simulink model "shipp"  (R2016b)
settings: Solver=ode45  StartTime=0.0  StopTime=1000  RelTol=1e-3  EnableMultiTasking=on
values from neighbouring files (symbols this model uses):
  K = P_*data.Cd'*inv(data.Cd*P_*data.Cd'+data.R)    [Sfunctionshell.m]    (also in boatstuff.m = 0.1707)
  K_pd = 0.7647    [boatstuff.m]
  phi = 30    [boatstuff.m]
  T_d = T    (= 74.435)    [boatstuff.m]
  T_f = 8.391    [boatstuff.m]
libraries: simulink x4
settings Model: Creator=markh  LastModifiedBy=Kjetil
settings DataIOCC: LimitDataPoints=on  SaveFormat=Array  SignalLoggingSaveFormat=ModelDataLogs  SignalLoggingName=sigsOut
settings OptimizationCC: InitFltsAndDblsToZero=on  LifeSpan=inf
settings DebuggingCC: SaveWithParameterizedLinksMsg=none  UnderspecifiedInitializationDetection=Classic  MergeDetectMultiDrivingBlocksExec=none  SignalResolutionControl=TryResolveAllWithWarning  MultiTaskDSMMsg=warning  MultiTaskCondExecSysMsg=none  FcnCallInpInsideContextMsg=warning  StateNameClashWarn=warning  SFUnexpectedBacktrackingDiag=warning  SFNoUnconditionalDefaultTransitionDiag=warning  SFExecutionAtInitializationDiag=none
settings HardwareCC: ProdBitPerPointer=32  ProdBitPerSizeT=32  ProdBitPerPtrDiffT=32  ProdLargestAtomicFloat=None  ProdIntDivRoundTo=Undefined  ProdEndianess=Unspecified  ProdWordSize=32  ProdHWDeviceType=32-bit Generic  TargetUnknown=on
settings ModelReferenceCC: PropagateSignalLabelsOutOfModel=off
settings GRTTargetCC: TargetFcnLib=ansi_tfl_tmw.mat  TargetLangStandard=C89/C90 (ANSI)  GeneratePreprocessorConditionals=Disable all  CombineOutputUpdateFcns=off  GRTInterface=on
settings ConfigComp: CovMetricSettings=dw  CovHtmlReporting=on  CovSaveCumulativeToWorkspaceVar=on  CovSaveSingleToWorkspaceVar=on  CovExternalEMLEnable=off

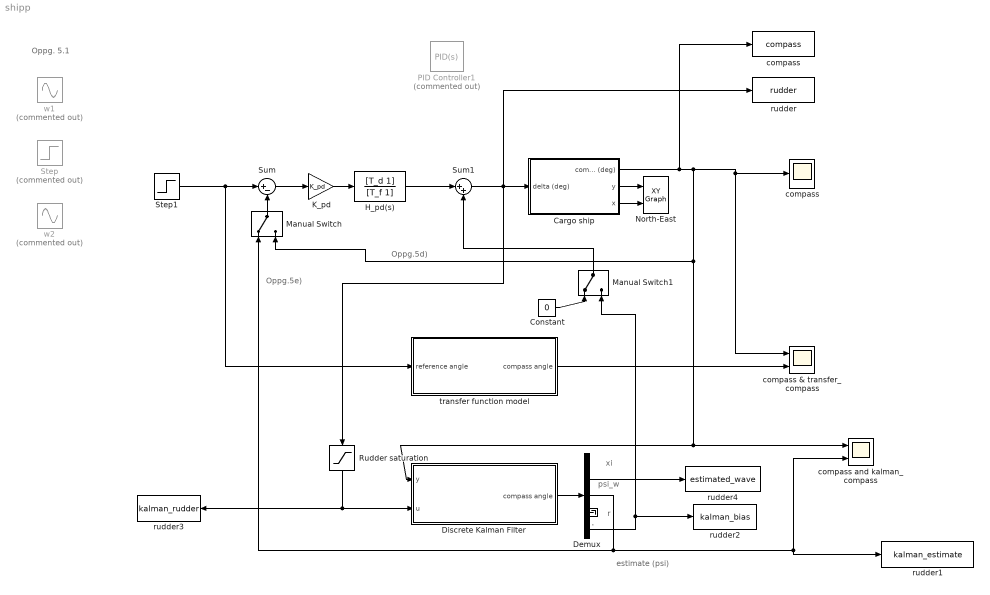
== system shipp ==
  note: Oppg.5d)
  note: Oppg.5e)
  note: r
  note: psi_w
  note: xi
  note: estimate (psi)
  note: Oppg. 5.1
  " H_pd(s)" : TransferFcn  Numerator=[T_d 1]  Denominator=[T_f 1]
  . : Terminator
  Cargo ship : Subsystem  mask(Simple shipmodel for a cargo ship){noise=on, current=on, logic=on}
      mask prompts: noise "measurement noise"; logic "waves"
      mask help:
      | Measurement noise:
      | 	checked = noise on
      | 	unchecked = noise off
      |
      | Current:
      | 	checked = current on
      | 	unchecked = current off
      |
      | Waves:
      | 	checked = waves on
      | 	unchecked = waves off
      |
      | Author: Jørgen Spjøtvold, 9/10-2003
      | TTK 4115 Linear system theory.
      | Modified by Jostein Bakkeheim 26/10-2006
  Constant : Constant  Value=0
  Demux : Demux  Outputs=5
  Discrete Kalman Filter : Subsystem
  K_pd : Gain  Gain=K_pd
  Manual Switch : ManualSwitch
  Manual Switch1 : ManualSwitch
  North-East : simulink/Sinks/XY Graph  xmin=-5000  xmax=5000  ymin=-5000  ymax=5000  st=-1
  PID Controller1 : simulink/Continuous/PID Controller  Commented=on  Controller=PID  TimeDomain=Continuous-time  SampleTime=-1  IntegratorMethod=Forward Euler  FilterMethod=Forward Euler  Form=Parallel  UseFilter=on  ControllerParametersSource=internal  P=0.0879832562005669  I=0.000147500393517768  D=7.30622580756413  N=0.0302786606051885  InitialConditionSource=internal  InitialConditionForIntegrator=0  InitialConditionForFilter=0  ExternalReset=none  LimitOutput=off  UpperSaturationLimit=inf  LowerSaturationLimit=-inf  LinearizeAsGain=on  AntiWindupMode=none  Kb=1  TrackingMode=off  Kt=1  PParamMin=[]  PParamMax=[]  IParamMin=[]  IParamMax=[]  DParamMin=[]  DParamMax=[]  NParamMin=[]  NParamMax=[]  KbParamMin=[]  KbParamMax=[]  KtParamMin=[]  KtParamMax=[]  POutMin=[]  POutMax=[]  IOutMin=[]  IOutMax=[]  DOutMin=[]  DOutMax=[]  NOutMin=[]  NOutMax=[]  KbOutMin=[]  KbOutMax=[]  KtOutMin=[]  KtOutMax=[]  IntegratorOutMin=[]  IntegratorOutMax=[]  FilterOutMin=[]  FilterOutMax=[]  SumOutMin=[]  SumOutMax=[]  SumI1OutMin=[]  SumI1OutMax=[]  SumI2OutMin=[]  SumI2OutMax=[]  SumI3OutMin=[]  SumI3OutMax=[]  SumDOutMin=[]  SumDOutMax=[]  SaturationOutMin=[]  SaturationOutMax=[]  IntegratorContinuousStateAttributes=''  IntegratorStateMustResolveToSignalObject=off  IntegratorRTWStateStorageClass=Auto  FilterContinuousStateAttributes=''  FilterStateMustResolveToSignalObject=off  FilterRTWStateStorageClass=Auto  DifferentiatorICPrevScaledInput=0  DifferentiatorOutMin=[]  DifferentiatorOutMax=[]
  Rudder saturation : Saturate  UpperLimit=45  LowerLimit=-45
  Step : Step  Commented=on  SampleTime=0
  Step1 : Step  Time=0  After=phi  SampleTime=0
  Sum : Sum  Inputs=|+-
  Sum1 : Sum  Inputs=|++
  compass : ToWorkspace  VariableName=compass  SaveFormat=Timeseries  SampleTime=-1
  "compass " : Scope
  compass & transfer_compass : Scope  NumInputPorts=2
  compass and kalman_compass : Scope  NumInputPorts=2
  rudder : ToWorkspace  VariableName=rudder  SaveFormat=Timeseries  SampleTime=-1
  rudder1 : ToWorkspace  VariableName=kalman_estimate  SaveFormat=Timeseries  SampleTime=-1
  rudder2 : ToWorkspace  VariableName=kalman_bias  SaveFormat=Timeseries  SampleTime=-1
  rudder3 : ToWorkspace  VariableName=kalman_rudder  SaveFormat=Timeseries  SampleTime=-1
  rudder4 : ToWorkspace  VariableName=estimated_wave  SaveFormat=Timeseries  SampleTime=-1
  transfer function model : Subsystem
  "w1 " : Sin  Commented=on  Frequency=0.005  SampleTime=0
  w2 : Sin  Commented=on  Frequency=0.05  SampleTime=0
  wires:
  Cargo ship/3(x) -> North-East/2
  Cargo ship/2(y) -> North-East/1
  Step1/1 -> Sum/1, transfer function model/1(reference angle)
  Sum/1 -> K_pd/1
  K_pd/1 -> " H_pd(s)"/1
  transfer function model/1(compass angle) -> compass & transfer_compass/2
  Discrete Kalman Filter/1(compass angle) -> Demux/1
  Sum1/1 -> Rudder saturation/1, rudder/1, Cargo ship/1(delta (deg))
  Demux/3 -> Manual Switch/1, compass and kalman_compass/2, rudder1/1
  Cargo ship/1(compass (deg)) -> compass/1, Manual Switch/2, Discrete Kalman Filter/1(y), compass and kalman_compass/1, "compass "/1, compass & transfer_compass/1
  Demux/4 -> ./1
  Manual Switch/1 -> Sum/2
  Manual Switch1/1 -> Sum1/2
  Constant/1 -> Manual Switch1/1
  Demux/5 -> Manual Switch1/2, rudder2/1
  " H_pd(s)"/1 -> Sum1/1
  Rudder saturation/1 -> rudder3/1, Discrete Kalman Filter/2(u)
  Demux/2 -> rudder4/1

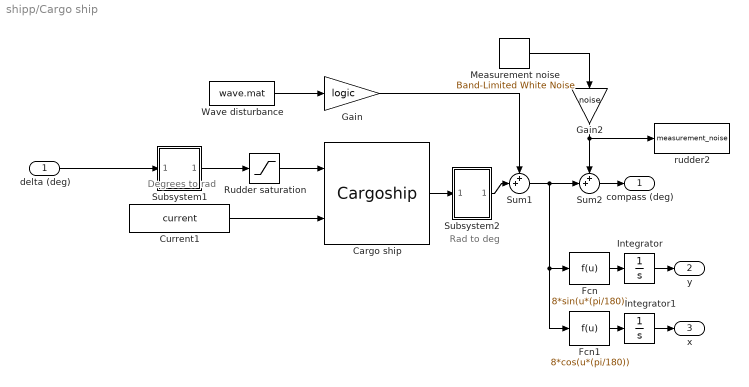
== system shipp/Cargo ship ==
  note: Degrees to rad
  note: Rad to deg
  delta (deg) : Inport
  Cargo ship : S-Function  FunctionName=Cargoship  SFunctionDeploymentMode=off  EnableBusSupport=off  mask(Cargo ship){}
      mask help:
      | S-function which simulates a cargo ship.
      |
      | Author: Jørgen Spjøtvold
      | 20.10-2003
      | Modified by Jostein Bakkeheim 27.10.2006
  Current1 : Constant  Value=current
  Fcn : Fcn  Expr=8*sin(u*(pi/180))
  Fcn1 : Fcn  Expr=8*cos(u*(pi/180))
  Gain : Gain  Gain=logic  SaturateOnIntegerOverflow=on  OutDataTypeStr=Inherit: Same as input  ParamDataTypeStr=Inherit: Same as input
  Gain2 : Gain  Gain=noise  SaturateOnIntegerOverflow=on  OutDataTypeStr=Inherit: Same as input  ParamDataTypeStr=Inherit: Same as input
  Integrator : Integrator
  Integrator1 : Integrator
  Measurement noise : simulink/Sources/Band-Limited White Noise  Cov=[0.001]  Ts=.5  seed=[23341]
  Rudder saturation : Saturate  UpperLimit=45*(pi/180)  LowerLimit=-45*(pi/180)
  Subsystem1 : Subsystem  mask(degrees to radians){}
      mask help: Converts degrees to radians
      mask Display: fprintf('D2R');
  Subsystem2 : Subsystem  mask(radians to degrees){}
      mask help: Converts radians to degrees
      mask Display: fprintf('R2D');
  Sum1 : Sum  Inputs=++|  SaturateOnIntegerOverflow=on
  Sum2 : Sum  Inputs=++|  SaturateOnIntegerOverflow=on
  Wave disturbance : FromFile  FileName=wave.mat  SampleTime=0
  rudder2 : ToWorkspace  VariableName=measurement_noise  SaveFormat=Timeseries  SampleTime=-1
  compass (deg) : Outport
  y : Outport  Port=2
  x : Outport  Port=3
  wires:
  delta (deg)/1 -> Subsystem1/1(In1)
  Fcn/1 -> Integrator/1
  Integrator/1 -> y/1
  Fcn1/1 -> Integrator1/1
  Integrator1/1 -> x/1
  Wave disturbance/1 -> Gain/1
  Subsystem2/1(Out1) -> Sum1/2
  Sum1/1 -> Fcn/1, Fcn1/1, Sum2/2
  Cargo ship/1 -> Subsystem2/1(In1)
  Subsystem1/1(Out1) -> Rudder saturation/1
  Rudder saturation/1 -> Cargo ship/1
  Sum2/1 -> compass (deg)/1
  Measurement noise/1 -> Gain2/1
  Current1/1 -> Cargo ship/2
  Gain/1 -> Sum1/1
  Gain2/1 -> rudder2/1, Sum2/1

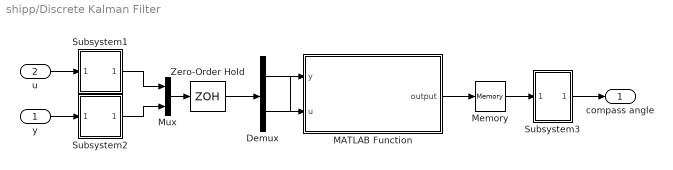
== system shipp/Discrete Kalman Filter ==
  y : Inport
  u : Inport  Port=2
  Demux : Demux  Outputs=2
  MATLAB Function : MATLAB Function  TreatAsAtomicUnit=on
  Memory : Memory
  Mux : Mux  Inputs=2
  Subsystem1 : Subsystem  mask(degrees to radians){}
      mask help: Converts degrees to radians
      mask Display: fprintf('D2R');
  Subsystem2 : Subsystem  mask(degrees to radians){}
      mask help: Converts degrees to radians
      mask Display: fprintf('D2R');
  Subsystem3 : Subsystem  mask(radians to degrees){}
      mask help: Converts radians to degrees
      mask Display: fprintf('R2D');
  Zero-Order Hold : ZeroOrderHold  SampleTime=0.1
  compass angle : Outport
  wires:
  Mux/1 -> Zero-Order Hold/1
  Zero-Order Hold/1 -> Demux/1
  Demux/1 -> MATLAB Function/2(u)
  Demux/2 -> MATLAB Function/1(y)
  MATLAB Function/1(output) -> Memory/1
  u/1 -> Subsystem1/1(In1)
  Subsystem1/1(Out1) -> Mux/1
  Subsystem2/1(Out1) -> Mux/2
  y/1 -> Subsystem2/1(In1)
  Subsystem3/1(Out1) -> compass angle/1
  Memory/1 -> Subsystem3/1(In1)

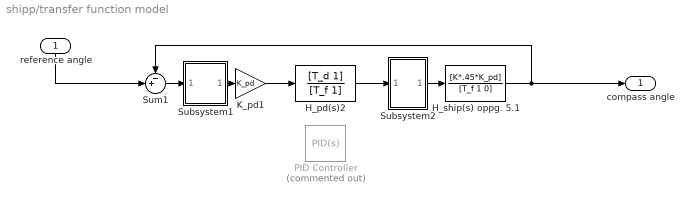
== system shipp/transfer function model ==
  reference angle : Inport
  " H_pd(s)2" : TransferFcn  Numerator=[T_d 1]  Denominator=[T_f 1]
  H_ship(s) oppg. 5.1 : TransferFcn  Numerator=[K*.45*K_pd]  Denominator=[T_f 1 0]
  K_pd1 : Gain  Gain=K_pd
  PID Controller : simulink/Continuous/PID Controller  Commented=on  Controller=PID  TimeDomain=Continuous-time  SampleTime=-1  IntegratorMethod=Forward Euler  FilterMethod=Forward Euler  Form=Parallel  UseFilter=on  ControllerParametersSource=internal  P=1.86157451877721  I=0.0260079579913027  D=13.0101900287485  N=0.0884818072308436  InitialConditionSource=internal  InitialConditionForIntegrator=0  InitialConditionForFilter=0  ExternalReset=none  LimitOutput=off  UpperSaturationLimit=inf  LowerSaturationLimit=-inf  LinearizeAsGain=on  AntiWindupMode=none  Kb=1  TrackingMode=off  Kt=1  PParamMin=[]  PParamMax=[]  IParamMin=[]  IParamMax=[]  DParamMin=[]  DParamMax=[]  NParamMin=[]  NParamMax=[]  KbParamMin=[]  KbParamMax=[]  KtParamMin=[]  KtParamMax=[]  POutMin=[]  POutMax=[]  IOutMin=[]  IOutMax=[]  DOutMin=[]  DOutMax=[]  NOutMin=[]  NOutMax=[]  KbOutMin=[]  KbOutMax=[]  KtOutMin=[]  KtOutMax=[]  IntegratorOutMin=[]  IntegratorOutMax=[]  FilterOutMin=[]  FilterOutMax=[]  SumOutMin=[]  SumOutMax=[]  SumI1OutMin=[]  SumI1OutMax=[]  SumI2OutMin=[]  SumI2OutMax=[]  SumI3OutMin=[]  SumI3OutMax=[]  SumDOutMin=[]  SumDOutMax=[]  SaturationOutMin=[]  SaturationOutMax=[]  IntegratorContinuousStateAttributes=''  IntegratorStateMustResolveToSignalObject=off  IntegratorRTWStateStorageClass=Auto  FilterContinuousStateAttributes=''  FilterStateMustResolveToSignalObject=off  FilterRTWStateStorageClass=Auto  DifferentiatorICPrevScaledInput=0  DifferentiatorOutMin=[]  DifferentiatorOutMax=[]
  Subsystem1 : Subsystem  mask(degrees to radians){}
      mask help: Converts degrees to radians
      mask Display: fprintf('D2R');
  Subsystem2 : Subsystem  mask(radians to degrees){}
      mask help: Converts radians to degrees
      mask Display: fprintf('R2D');
  Sum1 : Sum  Inputs=-+|
  compass angle : Outport
  wires:
  reference angle/1 -> Sum1/2
  K_pd1/1 -> " H_pd(s)2"/1
  Subsystem1/1(Out1) -> K_pd1/1
  Sum1/1 -> Subsystem1/1(In1)
  H_ship(s) oppg. 5.1/1 -> compass angle/1, Sum1/1
  Subsystem2/1(Out1) -> H_ship(s) oppg. 5.1/1
  " H_pd(s)2"/1 -> Subsystem2/1(In1)

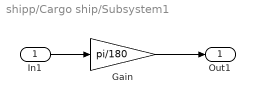
== system shipp/Cargo ship/Subsystem1 ==
  In1 : Inport
  Gain : Gain  Gain=pi/180  SaturateOnIntegerOverflow=on  OutDataTypeStr=Inherit: Same as input  ParamDataTypeStr=Inherit: Same as input
  Out1 : Outport
  wires:
  Gain/1 -> Out1/1
  In1/1 -> Gain/1

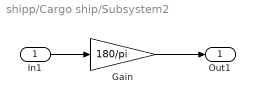
== system shipp/Cargo ship/Subsystem2 ==
  In1 : Inport
  Gain : Gain  Gain=180/pi  SaturateOnIntegerOverflow=on  OutDataTypeStr=Inherit: Same as input  ParamDataTypeStr=Inherit: Same as input
  Out1 : Outport
  wires:
  Gain/1 -> Out1/1
  In1/1 -> Gain/1

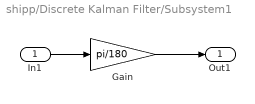
== system shipp/Discrete Kalman Filter/Subsystem1 ==
  In1 : Inport
  Gain : Gain  Gain=pi/180  SaturateOnIntegerOverflow=on  OutDataTypeStr=Inherit: Same as input  ParamDataTypeStr=Inherit: Same as input
  Out1 : Outport
  wires:
  Gain/1 -> Out1/1
  In1/1 -> Gain/1

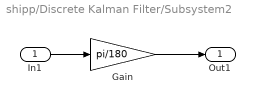
== system shipp/Discrete Kalman Filter/Subsystem2 ==
  In1 : Inport
  Gain : Gain  Gain=pi/180  SaturateOnIntegerOverflow=on  OutDataTypeStr=Inherit: Same as input  ParamDataTypeStr=Inherit: Same as input
  Out1 : Outport
  wires:
  Gain/1 -> Out1/1
  In1/1 -> Gain/1

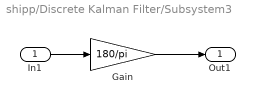
== system shipp/Discrete Kalman Filter/Subsystem3 ==
  In1 : Inport
  Gain : Gain  Gain=180/pi  SaturateOnIntegerOverflow=on  OutDataTypeStr=Inherit: Same as input  ParamDataTypeStr=Inherit: Same as input
  Out1 : Outport
  wires:
  Gain/1 -> Out1/1
  In1/1 -> Gain/1

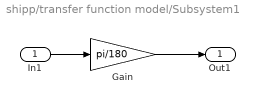
== system shipp/transfer function model/Subsystem1 ==
  In1 : Inport
  Gain : Gain  Gain=pi/180  SaturateOnIntegerOverflow=on  OutDataTypeStr=Inherit: Same as input  ParamDataTypeStr=Inherit: Same as input
  Out1 : Outport
  wires:
  Gain/1 -> Out1/1
  In1/1 -> Gain/1

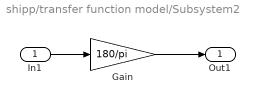
== system shipp/transfer function model/Subsystem2 ==
  In1 : Inport
  Gain : Gain  Gain=180/pi  SaturateOnIntegerOverflow=on  OutDataTypeStr=Inherit: Same as input  ParamDataTypeStr=Inherit: Same as input
  Out1 : Outport
  wires:
  Gain/1 -> Out1/1
  In1/1 -> Gain/1

== matlab function shipp/Discrete Kalman Filter/MATLAB Function ==
  data: y input; u input; output output; model_struct parameter
function output = DiscreteKalman( y, u, model_struct)
%DISCRETEKALMAN 
%   - MATLAB function implementation of a discrete Kalman filter -

persistent init_flag P_pri x_est_pri
Ad = model_struct.Ad;
Bd = model_struct.Bd;
Ed = model_struct.Ed;
Cd = model_struct.Cd;
Q = model_struct.Q;
R = model_struct.R;
I = model_struct.I;

if isempty(init_flag)
    init_flag = 1;
    x_0_est_pri = [0;0;0;0;0];
    P_0_pri = [1 0 0 0 0;
             0 0.13 0 0 0;
             0 0 pi^2 0 0;
             0 0 0 1 0;
             0 0 0 0 2.5*10^(-4)];
    P_pri = P_0_pri;
    x_est_pri = x_0_est_pri;
end

% Kalman gain
L = P_pri * Cd' * inv(Cd * P_pri * Cd' + R);

% Update estimate
x_est_post = x_est_pri + L * (y - Cd * x_est_pri);

% Update error cov. matrix
P = (I - L*Cd) * P_pri * (I - L*Cd)' + L * R * L';

x_est_next_pri = Ad * x_est_post + Bd*u;
P_next_pri = Ad*P*Ad' + Ed*Q*Ed';

x_est_pri = x_est_next_pri;
P_pri = P_next_pri;

output = [x_est_post];
end
